simulink model "decoderN4"  (R2016b)
settings: Solver=FixedStepDiscrete  StartTime=0.0  StopTime=10.0  RelTol=1e-3
libraries: simulink x13
settings Model: DataTypeOverride=Off  Creator=hasee  LastModifiedBy=hasee
settings DataIOCC: LimitDataPoints=on  SaveOutput=off  SaveTime=off
settings OptimizationCC: BlockReduction=off  ConditionallyExecuteInputs=off  DefaultParameterBehavior=Inlined  LifeSpan=inf
settings DebuggingCC: AlgebraicLoopMsg=error  SingleTaskRateTransMsg=error  AllowSymbolicDim=off  StrictBusMsg=ErrorOnBusTreatedAsVector  SFUnexpectedBacktrackingDiag=warning  SFNoUnconditionalDefaultTransitionDiag=warning  SFExecutionAtInitializationDiag=none
settings HardwareCC: ProdBitPerPointer=32  ProdBitPerSizeT=32  ProdBitPerPtrDiffT=32  ProdLargestAtomicFloat=None  ProdIntDivRoundTo=Undefined  ProdEndianess=Unspecified  ProdWordSize=32  ProdHWDeviceType=ASIC/FPGA->ASIC/FPGA  ProdEqTarget=off
settings GRTTargetCC: TargetLangStandard=C89/C90 (ANSI)  GeneratePreprocessorConditionals=Disable all
settings ConfigComp: CovScope=ReferencedModels  CovMetricSettings=dw  CovHtmlReporting=on  CovSaveCumulativeToWorkspaceVar=on  CovSaveSingleToWorkspaceVar=on  CovExternalEMLEnable=off  CovSFcnEnable=off

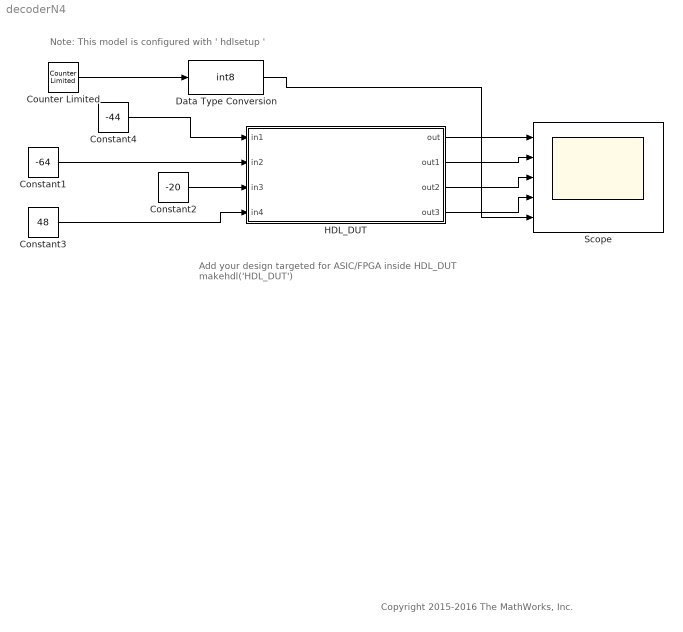
== system decoderN4 ==
  note: Note: This model is configured with ' hdlsetup '
  note: Add your design targeted for ASIC/FPGA inside HDL_DUT
      | makehdl('HDL_DUT')
  note: Copyright 2015-2016 The MathWorks, Inc.
  Constant1 : Constant  Value=-64  OutDataTypeStr=int8  SampleTime=-1
  Constant2 : Constant  Value=-20  OutDataTypeStr=int8  SampleTime=-1
  Constant3 : Constant  Value=48  OutDataTypeStr=int8  SampleTime=-1
  Constant4 : Constant  Value=-44  OutDataTypeStr=int8  SampleTime=-1
  Counter Limited : simulink/Sources/Counter Limited  uplimit=20  tsamp=-1
  Data Type Conversion : DataTypeConversion  OutDataTypeStr=int8
  HDL_DUT : Subsystem
  Scope : Scope  NumInputPorts=5
  wires:
  Counter Limited/1 -> Data Type Conversion/1
  HDL_DUT/1(out) -> Scope/1
  HDL_DUT/2(out1) -> Scope/2
  HDL_DUT/3(out2) -> Scope/3
  HDL_DUT/4(out3) -> Scope/4
  Constant1/1 -> HDL_DUT/2(in2)
  Constant3/1 -> HDL_DUT/4(in4)
  Constant2/1 -> HDL_DUT/3(in3)
  Data Type Conversion/1 -> Scope/5
  Constant4/1 -> HDL_DUT/1(in1)

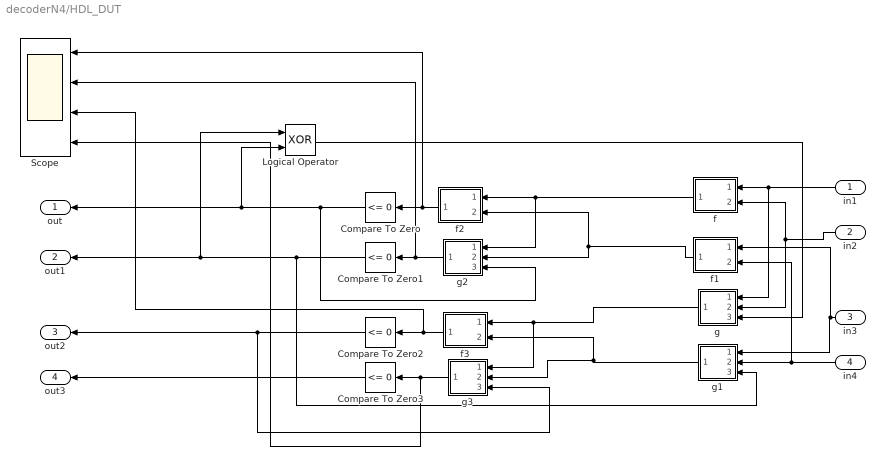
== system decoderN4/HDL_DUT ==
  in1 : Inport
  in2 : Inport  Port=2
  in3 : Inport  Port=3
  in4 : Inport  Port=4
  Compare To Zero{,1..3} (4 alike) : simulink/Logic and Bit Operations/Compare To Zero  relop=<=  OutDataTypeStr=boolean
  Logical Operator : Logic  Operator=XOR  AllPortsSameDT=off  OutDataTypeStr=boolean
  Scope : Scope  NumInputPorts=4
  f : Subsystem
  f1 : Subsystem
  f2 : Subsystem
  f3 : Subsystem
  g : Subsystem
  g1 : Subsystem
  g2 : Subsystem
  g3 : Subsystem
  out : Outport
  out1 : Outport  Port=2
  out2 : Outport  Port=3
  out3 : Outport  Port=4
  wires:
  in1/1 -> g/1(in1), f/1(in1)
  in2/1 -> f/2(in2), g/2(in2)
  f/1(out1) -> g2/1(in1), f2/1(in1)
  f1/1(out1) -> g2/2(in2), f2/2(in2)
  f2/1(out1) -> Scope/1, Compare To Zero/1
  Compare To Zero/1 -> g2/3(in3), Logical Operator/2, out/1
  g2/1(out) -> Scope/2, Compare To Zero1/1
  Compare To Zero1/1 -> g1/3(in3), Logical Operator/1, out1/1
  Logical Operator/1 -> g/3(in3)
  in3/1 -> f1/1(in1), g1/1(in1)
  in4/1 -> f1/2(in2), g1/2(in2)
  f3/1(out1) -> Scope/3, Compare To Zero2/1
  g/1(out) -> g3/1(in1), f3/1(in1)
  g1/1(out) -> g3/2(in2), f3/2(in2)
  Compare To Zero2/1 -> g3/3(in3), out2/1
  g3/1(out) -> Scope/4, Compare To Zero3/1
  Compare To Zero3/1 -> out3/1

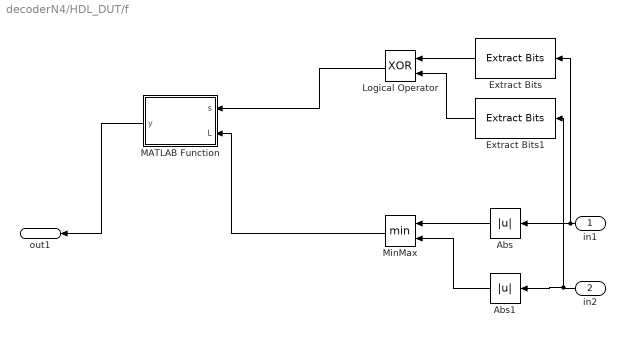
== system decoderN4/HDL_DUT/f ==
  in1 : Inport  OutDataTypeStr=int8
  in2 : Inport  Port=2  OutDataTypeStr=int8
  Abs : Abs
  Abs1 : Abs
  Extract Bits : simulink/Logic and Bit Operations/Extract Bits  bitsToExtract=Range starting with most significant bit  numBits=1  bitIdxRange=[0 ]  outScalingMode=Preserve fixed-point scaling
  Extract Bits1 : simulink/Logic and Bit Operations/Extract Bits  bitsToExtract=Range starting with most significant bit  numBits=1  bitIdxRange=[0 ]  outScalingMode=Preserve fixed-point scaling
  Logical Operator : Logic  Operator=XOR  AllPortsSameDT=off  OutDataTypeStr=boolean
  MATLAB Function : MATLAB Function  TreatAsAtomicUnit=on
  MinMax : MinMax  Inputs=2
  out1 : Outport
  wires:
  Extract Bits/1 -> Logical Operator/1
  in1/1 -> Abs/1, Extract Bits/1
  in2/1 -> Abs1/1, Extract Bits1/1
  Extract Bits1/1 -> Logical Operator/2
  Logical Operator/1 -> MATLAB Function/1(s)
  Abs/1 -> MinMax/1
  Abs1/1 -> MinMax/2
  MinMax/1 -> MATLAB Function/2(L)
  MATLAB Function/1(y) -> out1/1

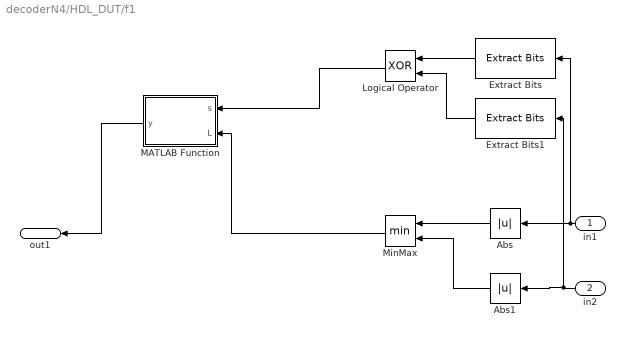
== system decoderN4/HDL_DUT/f1 ==
  in1 : Inport  OutDataTypeStr=int8
  in2 : Inport  Port=2  OutDataTypeStr=int8
  Abs : Abs
  Abs1 : Abs
  Extract Bits : simulink/Logic and Bit Operations/Extract Bits  bitsToExtract=Range starting with most significant bit  numBits=1  bitIdxRange=[0 ]  outScalingMode=Preserve fixed-point scaling
  Extract Bits1 : simulink/Logic and Bit Operations/Extract Bits  bitsToExtract=Range starting with most significant bit  numBits=1  bitIdxRange=[0 ]  outScalingMode=Preserve fixed-point scaling
  Logical Operator : Logic  Operator=XOR  AllPortsSameDT=off  OutDataTypeStr=boolean
  MATLAB Function : MATLAB Function  TreatAsAtomicUnit=on
  MinMax : MinMax  Inputs=2
  out1 : Outport
  wires:
  Extract Bits/1 -> Logical Operator/1
  in1/1 -> Abs/1, Extract Bits/1
  in2/1 -> Abs1/1, Extract Bits1/1
  Extract Bits1/1 -> Logical Operator/2
  Logical Operator/1 -> MATLAB Function/1(s)
  Abs/1 -> MinMax/1
  Abs1/1 -> MinMax/2
  MinMax/1 -> MATLAB Function/2(L)
  MATLAB Function/1(y) -> out1/1

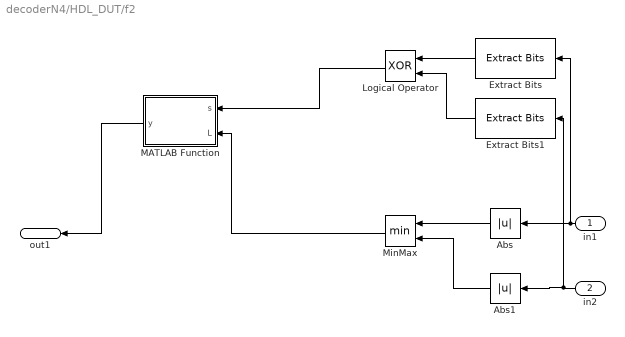
== system decoderN4/HDL_DUT/f2 ==
  in1 : Inport  OutDataTypeStr=int8
  in2 : Inport  Port=2  OutDataTypeStr=int8
  Abs : Abs
  Abs1 : Abs
  Extract Bits : simulink/Logic and Bit Operations/Extract Bits  bitsToExtract=Range starting with most significant bit  numBits=1  bitIdxRange=[0 ]  outScalingMode=Preserve fixed-point scaling
  Extract Bits1 : simulink/Logic and Bit Operations/Extract Bits  bitsToExtract=Range starting with most significant bit  numBits=1  bitIdxRange=[0 ]  outScalingMode=Preserve fixed-point scaling
  Logical Operator : Logic  Operator=XOR  AllPortsSameDT=off  OutDataTypeStr=boolean
  MATLAB Function : MATLAB Function  TreatAsAtomicUnit=on
  MinMax : MinMax  Inputs=2
  out1 : Outport
  wires:
  Extract Bits/1 -> Logical Operator/1
  in1/1 -> Abs/1, Extract Bits/1
  in2/1 -> Abs1/1, Extract Bits1/1
  Extract Bits1/1 -> Logical Operator/2
  Logical Operator/1 -> MATLAB Function/1(s)
  Abs/1 -> MinMax/1
  Abs1/1 -> MinMax/2
  MinMax/1 -> MATLAB Function/2(L)
  MATLAB Function/1(y) -> out1/1

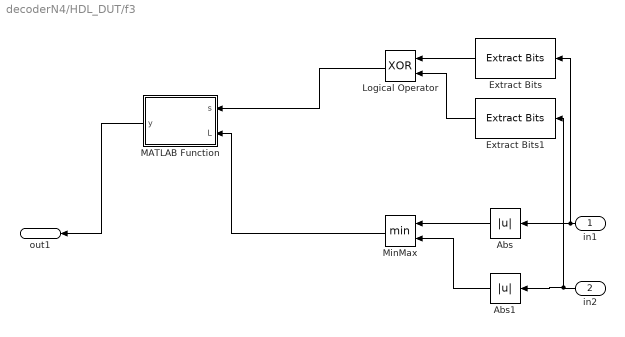
== system decoderN4/HDL_DUT/f3 ==
  in1 : Inport  OutDataTypeStr=int8
  in2 : Inport  Port=2  OutDataTypeStr=int8
  Abs : Abs
  Abs1 : Abs
  Extract Bits : simulink/Logic and Bit Operations/Extract Bits  bitsToExtract=Range starting with most significant bit  numBits=1  bitIdxRange=[0 ]  outScalingMode=Preserve fixed-point scaling
  Extract Bits1 : simulink/Logic and Bit Operations/Extract Bits  bitsToExtract=Range starting with most significant bit  numBits=1  bitIdxRange=[0 ]  outScalingMode=Preserve fixed-point scaling
  Logical Operator : Logic  Operator=XOR  AllPortsSameDT=off  OutDataTypeStr=boolean
  MATLAB Function : MATLAB Function  TreatAsAtomicUnit=on
  MinMax : MinMax  Inputs=2
  out1 : Outport
  wires:
  Extract Bits/1 -> Logical Operator/1
  in1/1 -> Abs/1, Extract Bits/1
  in2/1 -> Abs1/1, Extract Bits1/1
  Extract Bits1/1 -> Logical Operator/2
  Logical Operator/1 -> MATLAB Function/1(s)
  Abs/1 -> MinMax/1
  Abs1/1 -> MinMax/2
  MinMax/1 -> MATLAB Function/2(L)
  MATLAB Function/1(y) -> out1/1

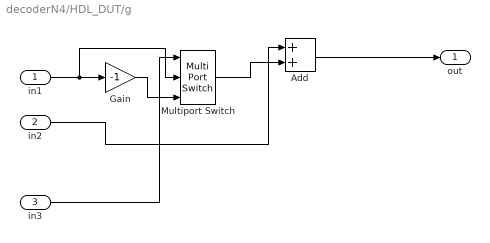
== system decoderN4/HDL_DUT/g ==
  in1 : Inport
  in2 : Inport  Port=2
  in3 : Inport  Port=3  OutDataTypeStr=boolean
  Add : Sum  Inputs=2  AccumDataTypeStr=int8
  Gain : Gain  Gain=-1  OutDataTypeStr=int8
  Multiport Switch : MultiPortSwitch  DataPortOrder=Zero-based contiguous  Inputs=2  OutDataTypeStr=int8
  out : Outport
  wires:
  in1/1 -> Multiport Switch/2, Gain/1
  in3/1 -> Multiport Switch/1
  Gain/1 -> Multiport Switch/3
  in2/1 -> Add/1
  Multiport Switch/1 -> Add/2
  Add/1 -> out/1

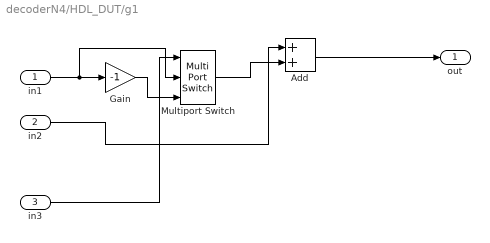
== system decoderN4/HDL_DUT/g1 ==
  in1 : Inport
  in2 : Inport  Port=2
  in3 : Inport  Port=3  OutDataTypeStr=boolean
  Add : Sum  Inputs=2  AccumDataTypeStr=int8
  Gain : Gain  Gain=-1  OutDataTypeStr=int8
  Multiport Switch : MultiPortSwitch  DataPortOrder=Zero-based contiguous  Inputs=2  OutDataTypeStr=int8
  out : Outport
  wires:
  in1/1 -> Multiport Switch/2, Gain/1
  in3/1 -> Multiport Switch/1
  Gain/1 -> Multiport Switch/3
  in2/1 -> Add/1
  Multiport Switch/1 -> Add/2
  Add/1 -> out/1

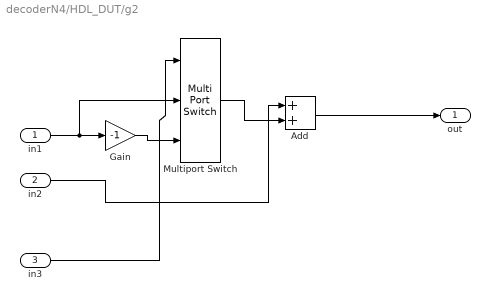
== system decoderN4/HDL_DUT/g2 ==
  in1 : Inport
  in2 : Inport  Port=2
  in3 : Inport  Port=3  OutDataTypeStr=boolean
  Add : Sum  Inputs=2  AccumDataTypeStr=int8
  Gain : Gain  Gain=-1  OutDataTypeStr=int8
  Multiport Switch : MultiPortSwitch  DataPortOrder=Zero-based contiguous  Inputs=2  OutDataTypeStr=int8
  out : Outport
  wires:
  in1/1 -> Multiport Switch/2, Gain/1
  in3/1 -> Multiport Switch/1
  Gain/1 -> Multiport Switch/3
  in2/1 -> Add/1
  Multiport Switch/1 -> Add/2
  Add/1 -> out/1

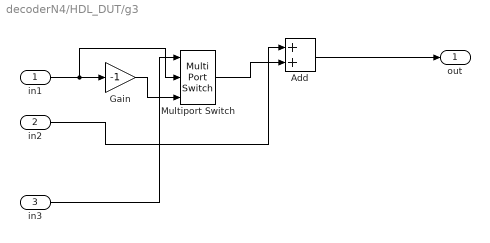
== system decoderN4/HDL_DUT/g3 ==
  in1 : Inport
  in2 : Inport  Port=2
  in3 : Inport  Port=3  OutDataTypeStr=boolean
  Add : Sum  Inputs=2  AccumDataTypeStr=int8
  Gain : Gain  Gain=-1  OutDataTypeStr=int8
  Multiport Switch : MultiPortSwitch  DataPortOrder=Zero-based contiguous  Inputs=2  OutDataTypeStr=int8
  out : Outport
  wires:
  in1/1 -> Multiport Switch/2, Gain/1
  in3/1 -> Multiport Switch/1
  Gain/1 -> Multiport Switch/3
  in2/1 -> Add/1
  Multiport Switch/1 -> Add/2
  Add/1 -> out/1

== matlab function decoderN4/HDL_DUT/f/MATLAB Function ==
  data: s input; y output; L input
function y = fcn(s,L)
%#codegen
if s ==1
    y = -L;
else
    y = L;
end

== matlab function decoderN4/HDL_DUT/f1/MATLAB Function ==
  data: s input; y output; L input
function y = fcn(s,L)
%#codegen
if s ==1
    y = -L;
else
    y = L;
end

== matlab function decoderN4/HDL_DUT/f2/MATLAB Function ==
  data: s input; y output; L input
function y = fcn(s,L)
%#codegen
if s ==1
    y = -L;
else
    y = L;
end

== matlab function decoderN4/HDL_DUT/f3/MATLAB Function ==
  data: s input; y output; L input
function y = fcn(s,L)
%#codegen
if s ==1
    y = -L;
else
    y = L;
end
